simulink model "simulacaoIsaque2"  (R2023a)
settings: Solver=VariableStepAuto  StartTime=0.0  StopTime=4  RelTol=1e-3
libraries: instrumentlib x2, cstblocks x1, simulink x1
settings Model: Creator=Aluno - LPR 3  LastModifiedBy=Aluno - LPR 4

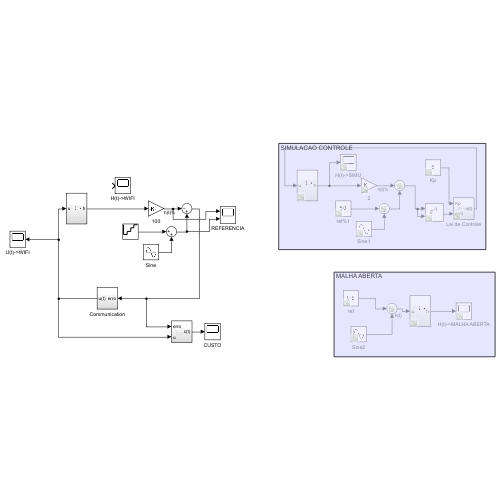
[thumbnail: Simulink's stored preview of the top-level diagram]
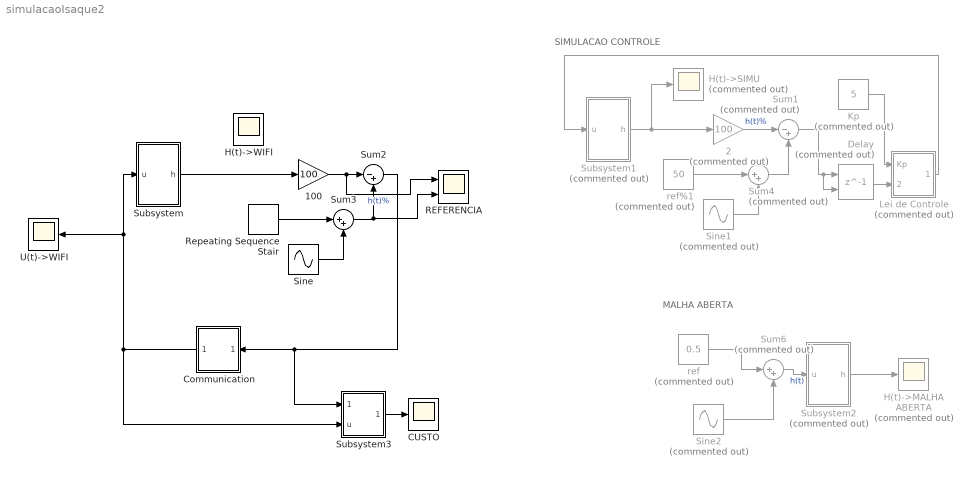
== system simulacaoIsaque2 ==
  note: SIMULACAO CONTROLE
  note: MALHA ABERTA
  100 : Gain  Gain=100
  2 : Gain  Commented=on  Gain=100
  CUSTO : Scope
  Communication : Subsystem
  Delay : Delay  Commented=on  DelayLength=1  InitialConditionSource=Input port  InitialCondition=0
      settings: InputPortMap=u0,p4
  H(t)->MALHA ABERTA : Scope  Commented=on
  H(t)->SIMU : Scope  Commented=on
  H(t)->WIFI : Scope
  Kp : Constant  Commented=on  Value=5
  Lei de Controle : Subsystem  Commented=on
  REFERENCIA : Scope  NumInputPorts=2
  Repeating Sequence Stair : simulink/Sources/Repeating Sequence Stair  OutValues=[20 40 60 80].'  tsamp=1  OutMin=[]  OutMax=[]  OutDataTypeStr=double  OutputDataTypeScalingMode=double  OutDataType=fixdt(0,8)  ConRadixGroup=Best Precision: Vector-wise  OutScaling=2^-12
  Sine : Sin  Frequency=20  SampleTime=0
  Sine1 : Sin  Commented=on  Amplitude=30  Frequency=4  SampleTime=0
  Sine2 : Sin  Commented=on  Amplitude=0.1  Frequency=4  SampleTime=0
  Subsystem : Subsystem
  Subsystem1 : Subsystem  Commented=on
  Subsystem2 : Subsystem  Commented=on
  Subsystem3 : Subsystem
  Sum1 : Sum  Commented=on  Inputs=|-+
  Sum2 : Sum  Inputs=|-+
  Sum3 : Sum  Inputs=|++
  Sum4 : Sum  Commented=on  Inputs=|++
  Sum6 : Sum  Commented=on  Inputs=|++
  U(t)->WIFI : Scope
  ref : Constant  Commented=on  Value=0.5
  ref%1 : Constant  Commented=on  Value=50
  wires:
  Repeating Sequence Stair/1 -> Sum3/1
  100/1 -> REFERENCIA/1, Sum2/1  "h(t)%"
  Sum3/1 -> Sum2/2, REFERENCIA/2
  Sine/1 -> Sum3/2
  Sum2/1 -> Subsystem3/1(erro), Communication/1(erro)
  Communication/1(u(t)) -> Subsystem/1(u), U(t)->WIFI/1, Subsystem3/2(u)
  Subsystem/1(h) -> 100/1
  Kp/1 -> Lei de Controle/1(Kp)
  2/1 -> Sum1/1  "h(t)%"
  Sum4/1 -> Sum1/2
  Sine1/1 -> Sum4/2
  ref%1/1 -> Sum4/1
  Subsystem1/1(h) -> H(t)->SIMU/1, 2/1
  Sum1/1 -> Delay/2, Delay/1
  Lei de Controle/1(u(t)) -> Subsystem1/1(u)
  Delay/1 -> Lei de Controle/2(erro)
  Subsystem2/1(h) -> H(t)->MALHA ABERTA/1
  ref/1 -> Sum6/1
  Sine2/1 -> Sum6/2
  Sum6/1 -> Subsystem2/1(u)  "h(t)"
  Subsystem3/1(c(t)) -> CUSTO/1

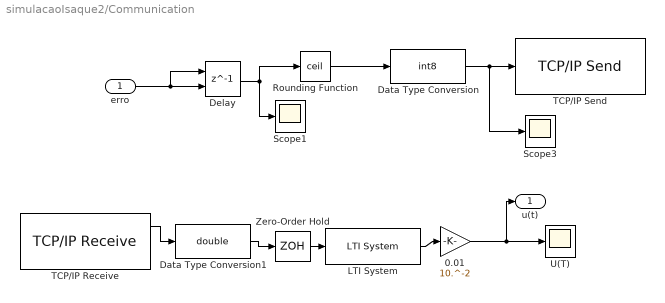
== system simulacaoIsaque2/Communication ==
  erro : Inport
  0.01 : Gain  Gain=10.^-2
  Data Type Conversion : DataTypeConversion  OutDataTypeStr=int8  SaturateOnIntegerOverflow=off  RndMeth=Floor
  Data Type Conversion1 : DataTypeConversion  OutDataTypeStr=double  SaturateOnIntegerOverflow=off  RndMeth=Floor
  Delay : Delay  DelayLength=1  InitialConditionSource=Input port  InitialCondition=0
      settings: InputPortMap=u0,p4
  LTI System : cstblocks/LTI System  sys=tf(1,[0.05 1])  IC=[]
  Rounding Function : Rounding  Operator=ceil
  Scope1 : Scope
  Scope3 : Scope
  TCP/IP Receive : instrumentlib/TCP//IP Receive  Host=192.168.4.1  Port=5000  DataSize=[ 1, 1 ]  DataType=uint8  ASCIIFormatting=%f  Terminator=CR  CustomTerminator=10  ByteOrder=big-endian  EnableBlockingMode=off  Timeout=10  SampleTime=0.0001  SimulateUsing=Interpreted execution
  TCP/IP Send : instrumentlib/TCP//IP Send  Host=192.168.4.1  Port=5000  ByteOrder=big-endian  EnableBlockingMode=off  Timeout=10  TransferDelay=on  SimulateUsing=Interpreted execution
  U(T) : Scope
  Zero-Order Hold : ZeroOrderHold  SampleTime=0.0001
  u(t) : Outport
  wires:
  Rounding Function/1 -> Data Type Conversion/1
  Delay/1 -> Rounding Function/1, Scope1/1
  0.01/1 -> u(t)/1, U(T)/1
  Data Type Conversion/1 -> Scope3/1, TCP/IP Send/1
  erro/1 -> Delay/1, Delay/2
  Zero-Order Hold/1 -> LTI System/1
  TCP/IP Receive/1 -> Data Type Conversion1/1
  Data Type Conversion1/1 -> Zero-Order Hold/1
  LTI System/1 -> 0.01/1

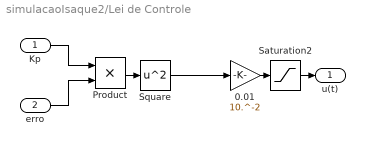
== system simulacaoIsaque2/Lei de Controle ==
  Kp : Inport
  erro : Inport  Port=2
  0.01 : Gain  Gain=10.^-2
  Product : Product
  Saturation2 : Saturate  UpperLimit=1  LowerLimit=0.000001
  Square : Math  Operator=square
  u(t) : Outport
  wires:
  Product/1 -> Square/1
  Kp/1 -> Product/1
  erro/1 -> Product/2
  Square/1 -> 0.01/1
  0.01/1 -> Saturation2/1
  Saturation2/1 -> u(t)/1

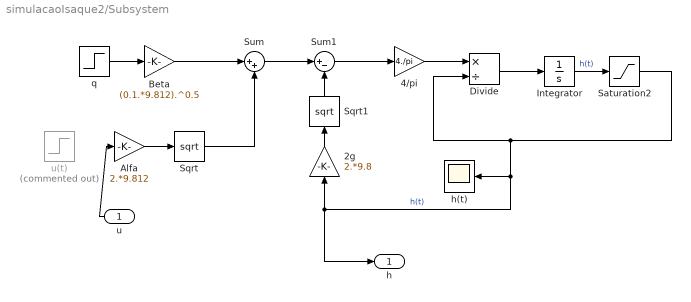
== system simulacaoIsaque2/Subsystem ==
  u : Inport
  2g : Gain  Gain=2.*9.8
  4/pi : Gain  Gain=4./pi
  Alfa : Gain  Gain=2.*9.812
  Beta : Gain  Gain=(0.1.*9.812).^0.5
  Divide : Product  Inputs=*/
  Integrator : Integrator  InitialCondition=0.1
  Saturation2 : Saturate  UpperLimit=1  LowerLimit=0.000000000001
  Sqrt : Sqrt
  Sqrt1 : Sqrt
  Sum : Sum  Inputs=|++
  Sum1 : Sum  Inputs=|+-
  h(t) : Scope
  q : Step  Time=0  After=0  SampleTime=0.1
  u(t) : Step  Commented=on  Time=0  Before=0.8  After=0.8  SampleTime=0.1
  h : Outport
  wires:
  Alfa/1 -> Sqrt/1
  Saturation2/1 -> Divide/2, h/1, 2g/1, h(t)/1  "h(t)"
  Sqrt1/1 -> Sum1/2
  4/pi/1 -> Divide/1
  2g/1 -> Sqrt1/1
  Sum/1 -> Sum1/1
  q/1 -> Beta/1
  Sqrt/1 -> Sum/2
  Divide/1 -> Integrator/1
  Sum1/1 -> 4/pi/1
  Beta/1 -> Sum/1
  Integrator/1 -> Saturation2/1  "h(t)"
  u/1 -> Alfa/1

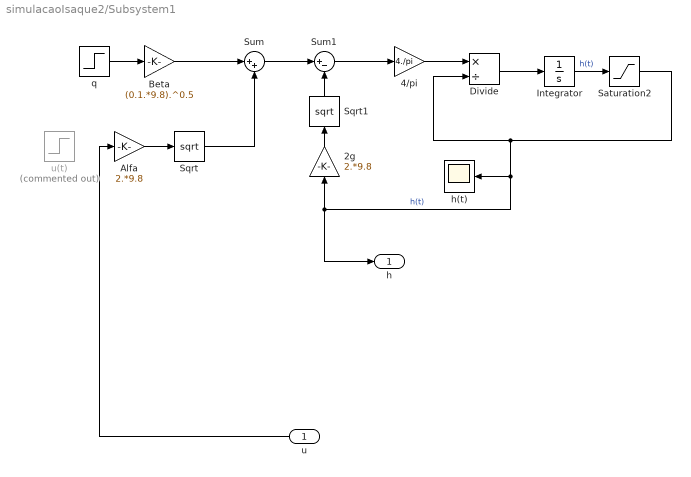
== system simulacaoIsaque2/Subsystem1 ==
  u : Inport
  2g : Gain  Gain=2.*9.8
  4/pi : Gain  Gain=4./pi
  Alfa : Gain  Gain=2.*9.8
  Beta : Gain  Gain=(0.1.*9.8).^0.5
  Divide : Product  Inputs=*/
  Integrator : Integrator  InitialCondition=0.1
  Saturation2 : Saturate  UpperLimit=1  LowerLimit=0.000000000001
  Sqrt : Sqrt
  Sqrt1 : Sqrt
  Sum : Sum  Inputs=|++
  Sum1 : Sum  Inputs=|+-
  h(t) : Scope
  q : Step  SampleTime=0.1
  u(t) : Step  Commented=on  Time=0  Before=0.8  After=0.8  SampleTime=0.1
  h : Outport
  wires:
  u/1 -> Alfa/1
  Integrator/1 -> Saturation2/1  "h(t)"
  Beta/1 -> Sum/1
  Sum1/1 -> 4/pi/1
  Divide/1 -> Integrator/1
  Sqrt/1 -> Sum/2
  q/1 -> Beta/1
  Sum/1 -> Sum1/1
  2g/1 -> Sqrt1/1
  4/pi/1 -> Divide/1
  Sqrt1/1 -> Sum1/2
  Saturation2/1 -> h(t)/1, 2g/1, h/1, Divide/2  "h(t)"
  Alfa/1 -> Sqrt/1

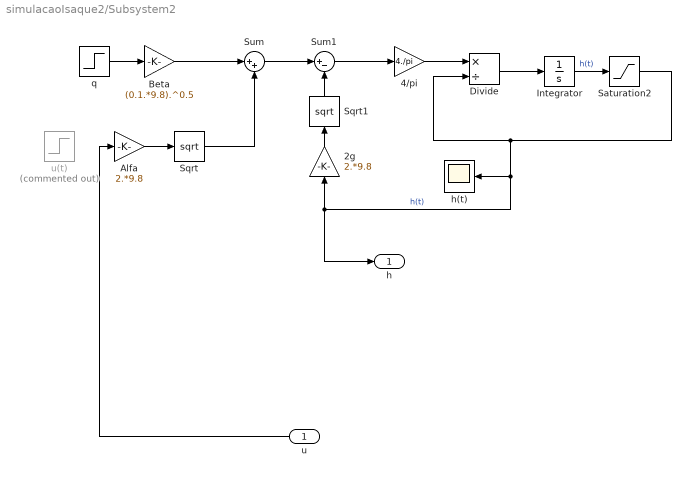
== system simulacaoIsaque2/Subsystem2 ==
  u : Inport
  2g : Gain  Gain=2.*9.8
  4/pi : Gain  Gain=4./pi
  Alfa : Gain  Gain=2.*9.8
  Beta : Gain  Gain=(0.1.*9.8).^0.5
  Divide : Product  Inputs=*/
  Integrator : Integrator  InitialCondition=0.1
  Saturation2 : Saturate  UpperLimit=1  LowerLimit=0.000000000001
  Sqrt : Sqrt
  Sqrt1 : Sqrt
  Sum : Sum  Inputs=|++
  Sum1 : Sum  Inputs=|+-
  h(t) : Scope
  q : Step  Time=0  After=0  SampleTime=0.1
  u(t) : Step  Commented=on  Time=0  Before=0.8  After=0.8  SampleTime=0.1
  h : Outport
  wires:
  Alfa/1 -> Sqrt/1
  Saturation2/1 -> Divide/2, h/1, 2g/1, h(t)/1  "h(t)"
  Sqrt1/1 -> Sum1/2
  4/pi/1 -> Divide/1
  2g/1 -> Sqrt1/1
  Sum/1 -> Sum1/1
  q/1 -> Beta/1
  Sqrt/1 -> Sum/2
  Divide/1 -> Integrator/1
  Sum1/1 -> 4/pi/1
  Beta/1 -> Sum/1
  Integrator/1 -> Saturation2/1  "h(t)"
  u/1 -> Alfa/1

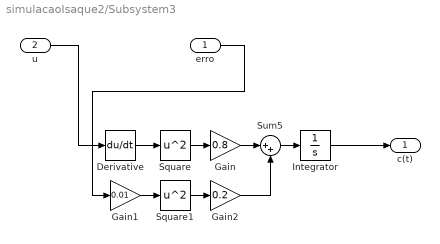
== system simulacaoIsaque2/Subsystem3 ==
  erro : Inport
  u : Inport  Port=2
  Derivative : Derivative
  Gain : Gain  Gain=0.8
  Gain1 : Gain  Gain=0.01
  Gain2 : Gain  Gain=0.2
  Integrator : Integrator
  Square : Math  Operator=square
  Square1 : Math  Operator=square
  Sum5 : Sum  Inputs=|++
  c(t) : Outport
  wires:
  Square1/1 -> Gain2/1
  Square/1 -> Gain/1
  Integrator/1 -> c(t)/1
  Gain/1 -> Sum5/1
  u/1 -> Derivative/1
  Sum5/1 -> Integrator/1
  Gain2/1 -> Sum5/2
  Gain1/1 -> Square1/1
  Derivative/1 -> Square/1
  erro/1 -> Gain1/1
